simulink model "hummer_solo"  (R2020b)
settings: Solver=VariableStepAuto  StartTime=0.0  StopTime=inf  RelTol=1e-3
libraries: simulink x1
settings Model: EnablePacing=on  Creator=kjartan  LastModifiedBy=kjartan

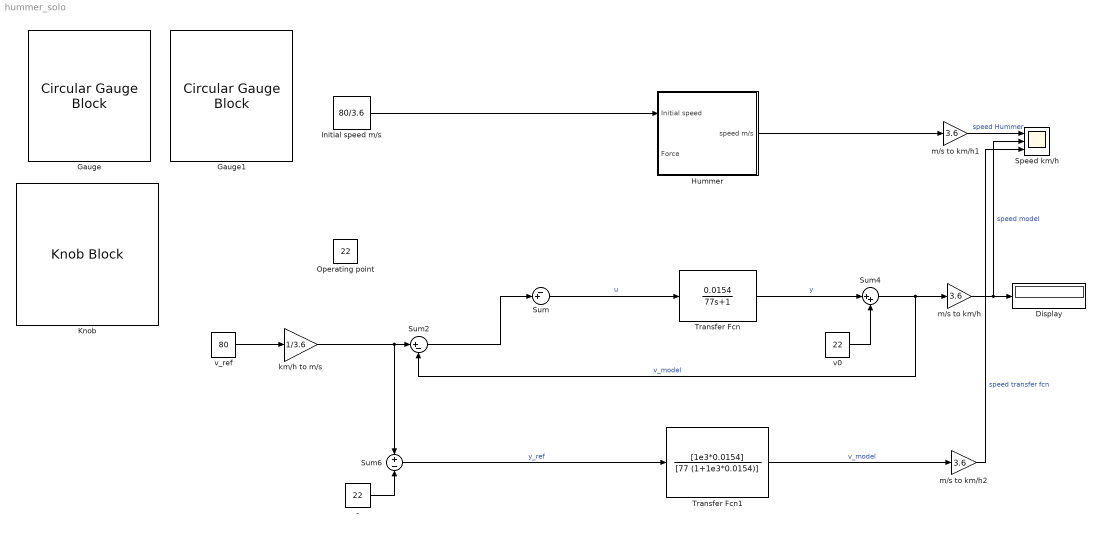
== system hummer_solo ==
  - : Constant  Value=22
  Display : Display
  Gauge : CircularGaugeBlock  ScaleMax=300  TickInterval=50
  Gauge1 : CircularGaugeBlock  ScaleMax=300  TickInterval=50
  Hummer : Subsystem
  Initial speed m/s : Constant  Value=80/3.6
  Knob : KnobBlock  ScaleMax=300  TickInterval=50
  Operating point : Constant  Value=22
  Speed km/h : Scope  NumInputPorts=3
  Sum : Sum  Inputs=-+|
  Sum2 : Sum  Inputs=|+-
  Sum4 : Sum  Inputs=|++
  Sum6 : Sum  Inputs=+|-
  Transfer Fcn : TransferFcn  Numerator=[0.0154]  Denominator=[77 1]
  Transfer Fcn1 : TransferFcn  Numerator=[1e3*0.0154]  Denominator=[77 (1+1e3*0.0154)]
  km/h to m/s : Gain  Gain=1/3.6
  m/s to km/h : Gain  Gain=3.6
  m/s to km/h1 : Gain  Gain=3.6
  m/s to km/h2 : Gain  Gain=3.6
  v0 : Constant  Value=22
  v_ref : Constant  Value=80
  wires:
  Sum/1 -> Transfer Fcn/1  "u"
  v0/1 -> Sum4/2
  Transfer Fcn/1 -> Sum4/1  "y"
  Sum4/1 -> m/s to km/h/1, Sum2/2  "v_model"
  Initial speed m/s/1 -> Hummer/1(Initial speed)
  Hummer/1(speed m/s) -> m/s to km/h1/1
  v_ref/1 -> km/h to m/s/1
  Sum2/1 -> Sum/2
  km/h to m/s/1 -> Sum6/1, Sum2/1
  m/s to km/h/1 -> Speed km/h/2, Display/1  "speed model"
  m/s to km/h1/1 -> Speed km/h/1  "speed Hummer"
  m/s to km/h2/1 -> Speed km/h/3  "speed transfer fcn"
  Transfer Fcn1/1 -> m/s to km/h2/1  "v_model"
  Sum6/1 -> Transfer Fcn1/1  "y_ref"
  -/1 -> Sum6/2

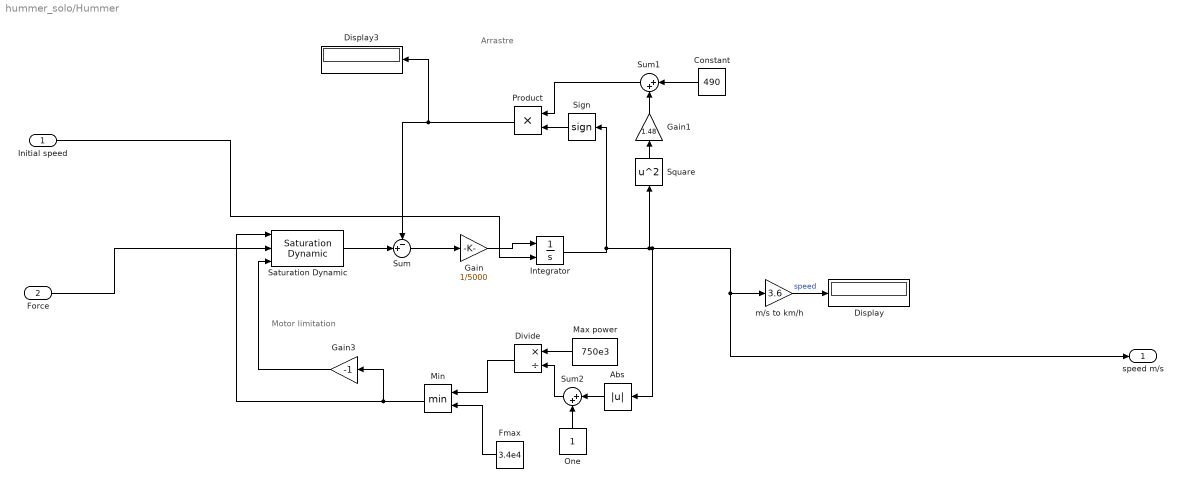
== system hummer_solo/Hummer ==
  note: Motor limitation
  note: Arrastre
  Initial speed : Inport
  Force : Inport  Port=2
  Abs : Abs
  Constant : Constant  Value=490
  Display : Display
  Display3 : Display
  Divide : Product  Inputs=*/
  Fmax : Constant  Value=3.4e4
  Gain : Gain  Gain=1/5000
  Gain1 : Gain  Gain=1.48
  Gain3 : Gain  Gain=-1
  Integrator : Integrator  InitialConditionSource=external
  Max power : Constant  Value=750e3
  Min : MinMax  Inputs=2
  One : Constant  OutDataTypeStr=Inherit: Inherit via back propagation
  Product : Product
  Saturation Dynamic : simulink/Discontinuities/Saturation Dynamic  OutMin=[]  OutMax=[]  OutDataTypeStr=Inherit: Same as second input  OutDataType=fixdt(1, 16)  OutScaling=2^-10  DoSatur=off
  Sign : Signum
  Square : Math  Operator=square  SaturateOnIntegerOverflow=on
  Sum : Sum  Inputs=-+|
  Sum1 : Sum  Inputs=|++
  Sum2 : Sum  Inputs=|++
  m/s to km/h : Gain  Gain=3.6
  speed m/s : Outport
  wires:
  Divide/1 -> Min/1
  Abs/1 -> Sum2/1
  Force/1 -> Saturation Dynamic/2
  m/s to km/h/1 -> Display/1  "speed"
  Square/1 -> Gain1/1
  Gain1/1 -> Sum1/2
  Sign/1 -> Product/2
  Constant/1 -> Sum1/1
  Sum/1 -> Gain/1
  Integrator/1 -> Abs/1, speed m/s/1, m/s to km/h/1, Square/1, Sign/1
  Sum1/1 -> Product/1
  Min/1 -> Gain3/1, Saturation Dynamic/1
  Initial speed/1 -> Integrator/2
  One/1 -> Sum2/2
  Fmax/1 -> Min/2
  Product/1 -> Sum/1, Display3/1
  Max power/1 -> Divide/1
  Gain/1 -> Integrator/1
  Gain3/1 -> Saturation Dynamic/3
  Saturation Dynamic/1 -> Sum/2
  Sum2/1 -> Divide/2
